simulink model "Deadlock_ACC"  (R2025a)
settings: Solver=VariableStepAuto  StartTime=0.0  StopTime=10.0  RelTol=1e-3
settings Model: Creator=nirmay  LastModifiedBy=nirmay

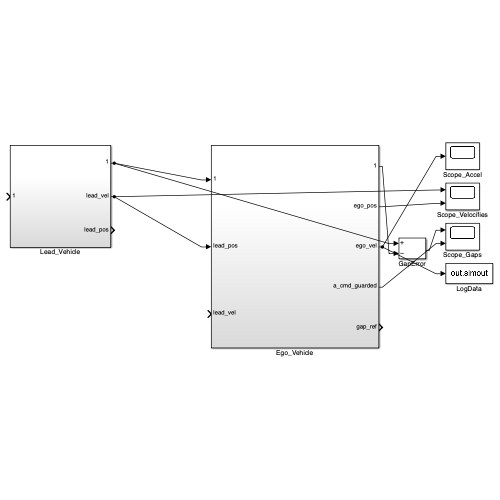
[thumbnail: Simulink's stored preview of the top-level diagram]
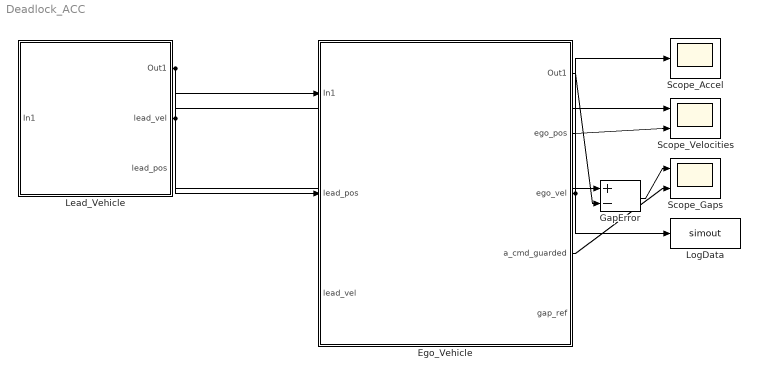
== system Deadlock_ACC ==
  Ego_Vehicle : Subsystem
  GapError : Sum  Inputs=+-
  Lead_Vehicle : Subsystem
  LogData : ToWorkspace  VariableName=simout  SaveFormat=Structure With Time  SampleTime=-1
  Scope_Accel : Scope
  Scope_Gaps : Scope  NumInputPorts=2
  Scope_Velocities : Scope  NumInputPorts=2
  wires:
  Lead_Vehicle/1(Out1) -> Ego_Vehicle/1(In1), GapError/1
  Lead_Vehicle/2(lead_vel) -> Ego_Vehicle/2(lead_pos), Scope_Velocities/1
  Ego_Vehicle/3(ego_vel) -> Scope_Accel/1, LogData/1
  Ego_Vehicle/2(ego_pos) -> Scope_Velocities/2
  Ego_Vehicle/1(Out1) -> GapError/2
  GapError/1 -> Scope_Gaps/1
  Ego_Vehicle/4(a_cmd_guarded) -> Scope_Gaps/2

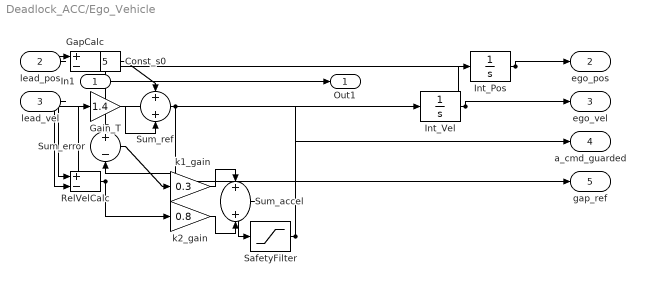
== system Deadlock_ACC/Ego_Vehicle ==
  In1 : Inport
  lead_pos : Inport  Port=2
  lead_vel : Inport  Port=3
  Const_s0 : Constant  Value=5
  Gain_T : Gain  Gain=1.4
  GapCalc : Sum  Inputs=+-
  Int_Pos : Integrator
  Int_Vel : Integrator
  RelVelCalc : Sum  Inputs=+-
  SafetyFilter : Saturate  UpperLimit=2  LowerLimit=-3
  Sum_accel : Sum
  Sum_error : Sum  Inputs=+-
  Sum_ref : Sum
  k1_gain : Gain  Gain=0.3
  k2_gain : Gain  Gain=0.8
  Out1 : Outport
  ego_pos : Outport  Port=2
  ego_vel : Outport  Port=3
  a_cmd_guarded : Outport  Port=4
  gap_ref : Outport  Port=5
  wires:
  In1/1 -> Out1/1
  lead_pos/1 -> GapCalc/1
  lead_vel/1 -> RelVelCalc/1
  Int_Pos/1 -> GapCalc/2, ego_pos/1
  Int_Vel/1 -> RelVelCalc/2, Int_Pos/1, ego_vel/1
  RelVelCalc/1 -> Gain_T/1, k2_gain/1
  Gain_T/1 -> Sum_ref/2
  Const_s0/1 -> Sum_ref/1
  Sum_ref/1 -> gap_ref/1, Sum_error/2
  GapCalc/1 -> Sum_error/1
  Sum_error/1 -> k1_gain/1
  k1_gain/1 -> Sum_accel/1
  k2_gain/1 -> Sum_accel/2
  Sum_accel/1 -> SafetyFilter/1
  SafetyFilter/1 -> Int_Vel/1, a_cmd_guarded/1

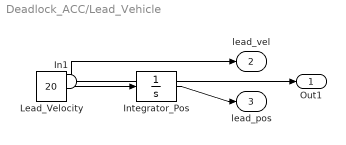
== system Deadlock_ACC/Lead_Vehicle ==
  In1 : Inport
  Integrator_Pos : Integrator  InitialCondition=40
  Lead_Velocity : Constant  Value=20
  Out1 : Outport
  lead_vel : Outport  Port=2
  lead_pos : Outport  Port=3
  wires:
  In1/1 -> Out1/1
  Lead_Velocity/1 -> Integrator_Pos/1, lead_vel/1
  Integrator_Pos/1 -> lead_pos/1
